simulink model "affine_single_integrator"  (R2020b)
settings: Solver=ode4  StartTime=0.0  StopTime=50  FixedStep=0.01  RelTol=1e-3
InitFcn:
  | Initial_Parameters;
values from neighbouring files (symbols this model uses):
  c_y = 0    [Initial_Parameters.m]
  delay = 0.01    [Initial_Parameters.m]    (also in run_by_script.m = 1)
  kalpha = 0.5    [Initial_Parameters.m]    (also in run_by_script.m = 4)
  kbeta = 1.5    [Initial_Parameters.m]    (also in run_by_script.m = 0.5)
  P0 = [2 0 ... (first row only)    [Initial_Parameters.m]    (also in run_by_script.m = [p(1,1:2:end)' p(2,2:2:end)'])
  stressMat = -fcn_StressMatrix(2,nodenum,m,P,neighborMat,fig_shape)    [Initial_Parameters.m]    (also in fcn_StressMatrix.m = -stressMat)
  vel_x = 0.1    [Initial_Parameters.m]
  vel_y = 0.5    [Initial_Parameters.m]
  w_y = 0.5    [Initial_Parameters.m]
settings Model: Creator=Fitz  LastModifiedBy=xpp
settings DebuggingCC: UnderSpecifiedDimensionMsg=warning

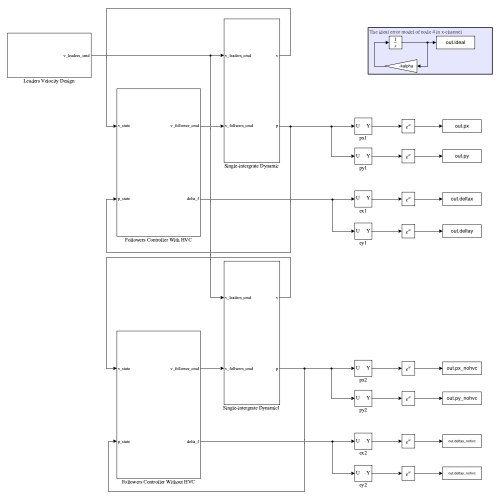
[thumbnail: Simulink's stored preview of the top-level diagram]
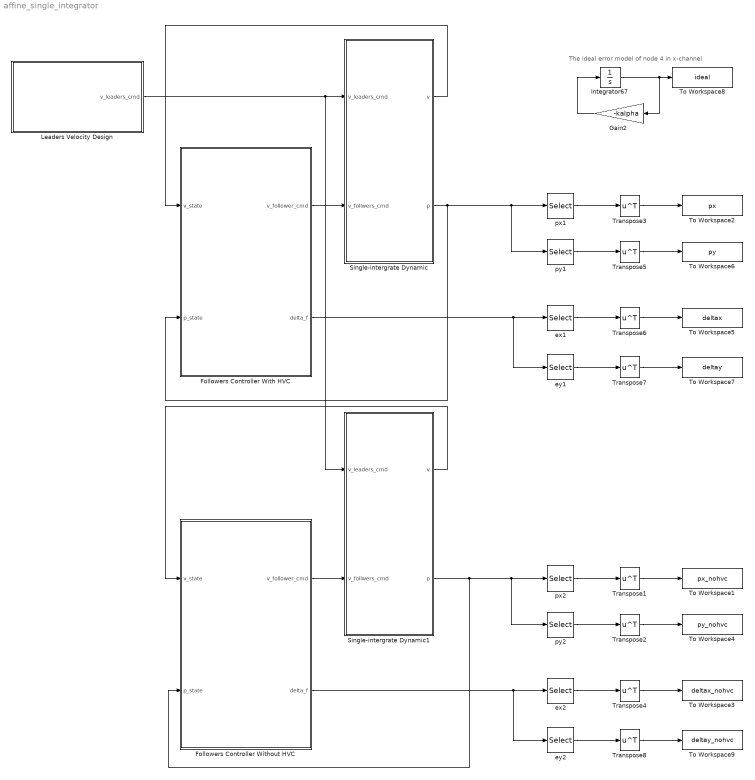
== system affine_single_integrator ==
  note: The ideal error model of node 4 in x-channel
  Followers Controller With HVC : Subsystem
  Followers Controller Without HVC : Subsystem
  Gain2 : Gain  Gain=-kalpha
  Integrator67 : Integrator  InitialCondition=P0(4,1)
  Leaders Velocity Design : Subsystem
  Single-intergrate Dynamic : Subsystem
  Single-intergrate Dynamic1 : Subsystem
  To Workspace1 : ToWorkspace  VariableName=px_nohvc  SampleTime=-1
      settings: Save2DSignal=2-D array (concatenate along first dimension)
  To Workspace2 : ToWorkspace  VariableName=px  SampleTime=-1
      settings: Save2DSignal=2-D array (concatenate along first dimension)
  To Workspace3 : ToWorkspace  VariableName=deltax_nohvc  SampleTime=-1
      settings: Save2DSignal=2-D array (concatenate along first dimension)
  To Workspace4 : ToWorkspace  VariableName=py_nohvc  SampleTime=-1
      settings: Save2DSignal=2-D array (concatenate along first dimension)
  To Workspace5 : ToWorkspace  VariableName=deltax  SampleTime=-1
      settings: Save2DSignal=2-D array (concatenate along first dimension)
  To Workspace6 : ToWorkspace  VariableName=py  SampleTime=-1
      settings: Save2DSignal=2-D array (concatenate along first dimension)
  To Workspace7 : ToWorkspace  VariableName=deltay  SampleTime=-1
      settings: Save2DSignal=2-D array (concatenate along first dimension)
  To Workspace8 : ToWorkspace  VariableName=ideal  SampleTime=-1
      settings: Save2DSignal=2-D array (concatenate along first dimension)
  To Workspace9 : ToWorkspace  VariableName=deltay_nohvc  SampleTime=-1
      settings: Save2DSignal=2-D array (concatenate along first dimension)
  Transpose{1..8} (8 alike) : Math  Operator=transpose  SaturateOnIntegerOverflow=on
  ex1 : Selector  NumberOfDimensions=2  InputPortWidth=3  IndexOptions=Select all,Index vector (dialog)  Indices=[1 3],1  OutputSizes=1,1
  ex2 : Selector  NumberOfDimensions=2  InputPortWidth=3  IndexOptions=Select all,Index vector (dialog)  Indices=[1 3],1  OutputSizes=1,1
  ey1 : Selector  NumberOfDimensions=2  InputPortWidth=3  IndexOptions=Select all,Index vector (dialog)  Indices=[1 3],2  OutputSizes=1,1
  ey2 : Selector  NumberOfDimensions=2  InputPortWidth=3  IndexOptions=Select all,Index vector (dialog)  Indices=[1 3],2  OutputSizes=1,1
  px1 : Selector  NumberOfDimensions=2  InputPortWidth=3  IndexOptions=Select all,Index vector (dialog)  Indices=[1 3],1  OutputSizes=1,1
  px2 : Selector  NumberOfDimensions=2  InputPortWidth=3  IndexOptions=Select all,Index vector (dialog)  Indices=[1 3],1  OutputSizes=1,1
  py1 : Selector  NumberOfDimensions=2  InputPortWidth=3  IndexOptions=Select all,Index vector (dialog)  Indices=[1 3],2  OutputSizes=1,1
  py2 : Selector  NumberOfDimensions=2  InputPortWidth=3  IndexOptions=Select all,Index vector (dialog)  Indices=[1 3],2  OutputSizes=1,1
  wires:
  Leaders Velocity Design/1(v_leaders_cmd) -> Single-intergrate Dynamic1/1(v_leaders_cmd), Single-intergrate Dynamic/1(v_leaders_cmd)
  Followers Controller With HVC/1(v_follower_cmd) -> Single-intergrate Dynamic/2(v_follwers_cmd)
  Single-intergrate Dynamic/1(v) -> Followers Controller With HVC/1(v_state)
  ey1/1 -> Transpose7/1
  py1/1 -> Transpose5/1
  Transpose3/1 -> To Workspace2/1
  Transpose7/1 -> To Workspace7/1
  Followers Controller With HVC/2(delta_f) -> ex1/1, ey1/1
  Transpose5/1 -> To Workspace6/1
  ex1/1 -> Transpose6/1
  Single-intergrate Dynamic/2(p) -> py1/1, px1/1, Followers Controller With HVC/2(p_state)
  Transpose6/1 -> To Workspace5/1
  px1/1 -> Transpose3/1
  Gain2/1 -> Integrator67/1
  Integrator67/1 -> To Workspace8/1, Gain2/1
  Followers Controller Without HVC/1(v_follower_cmd) -> Single-intergrate Dynamic1/2(v_follwers_cmd)
  Single-intergrate Dynamic1/1(v) -> Followers Controller Without HVC/1(v_state)
  Transpose1/1 -> To Workspace1/1
  ex2/1 -> Transpose4/1
  py2/1 -> Transpose2/1
  Followers Controller Without HVC/2(delta_f) -> ex2/1, ey2/1
  px2/1 -> Transpose1/1
  Transpose8/1 -> To Workspace9/1
  Transpose2/1 -> To Workspace4/1
  Transpose4/1 -> To Workspace3/1
  Single-intergrate Dynamic1/2(p) -> py2/1, px2/1, Followers Controller Without HVC/2(p_state)
  ey2/1 -> Transpose8/1

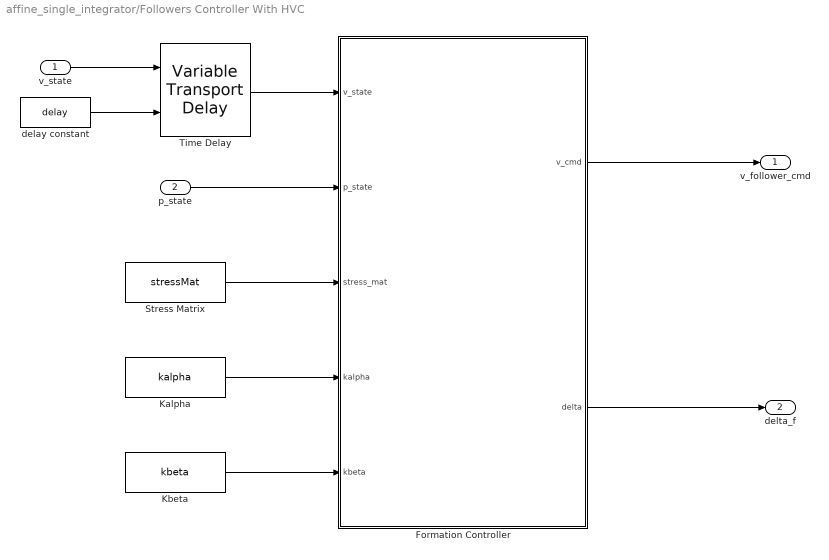
== system affine_single_integrator/Followers Controller With HVC ==
  v_state : Inport
  p_state : Inport  Port=2
  Formation Controller : MATLAB Function  TreatAsAtomicUnit=on
  Kalpha : Constant  Value=kalpha
  Kbeta : Constant  Value=kbeta
  Stress Matrix : Constant  Value=stressMat
  Time Delay : VariableTransportDelay  MaximumDelay=10
  delay constant : Constant  Value=delay
  v_follower_cmd : Outport
  delta_f : Outport  Port=2
  wires:
  delay constant/1 -> Time Delay/2
  v_state/1 -> Time Delay/1
  p_state/1 -> Formation Controller/2(p_state)
  Stress Matrix/1 -> Formation Controller/3(stress_mat)
  Kbeta/1 -> Formation Controller/5(kbeta)
  Kalpha/1 -> Formation Controller/4(kalpha)
  Formation Controller/1(v_cmd) -> v_follower_cmd/1
  Formation Controller/2(delta) -> delta_f/1
  Time Delay/1 -> Formation Controller/1(v_state)

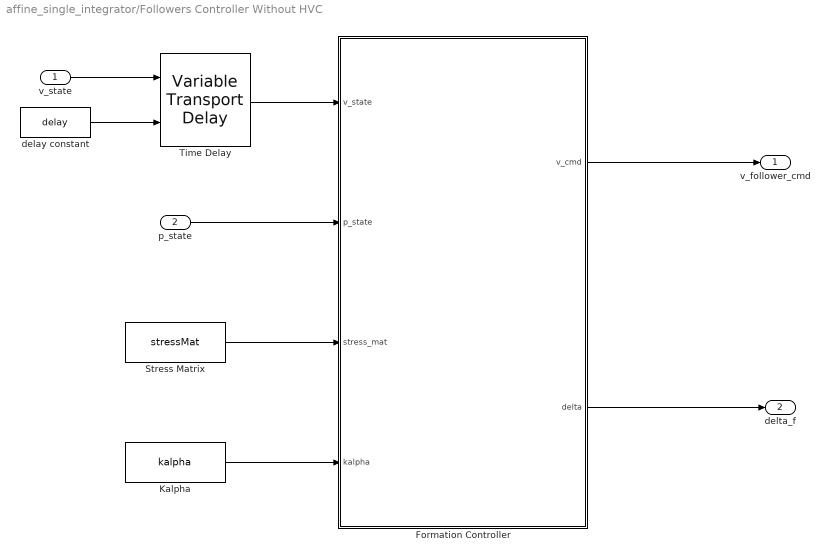
== system affine_single_integrator/Followers Controller Without HVC ==
  v_state : Inport
  p_state : Inport  Port=2
  Formation Controller : MATLAB Function  TreatAsAtomicUnit=on
  Kalpha : Constant  Value=kalpha
  Stress Matrix : Constant  Value=stressMat
  Time Delay : VariableTransportDelay  MaximumDelay=10
  delay constant : Constant  Value=delay
  v_follower_cmd : Outport
  delta_f : Outport  Port=2
  wires:
  delay constant/1 -> Time Delay/2
  v_state/1 -> Time Delay/1
  p_state/1 -> Formation Controller/2(p_state)
  Stress Matrix/1 -> Formation Controller/3(stress_mat)
  Kalpha/1 -> Formation Controller/4(kalpha)
  Formation Controller/1(v_cmd) -> v_follower_cmd/1
  Formation Controller/2(delta) -> delta_f/1
  Time Delay/1 -> Formation Controller/1(v_state)

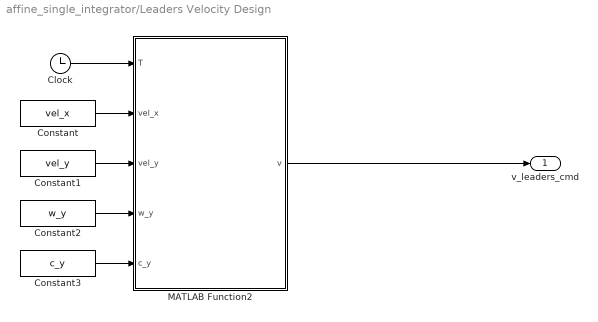
== system affine_single_integrator/Leaders Velocity Design ==
  Clock : Clock
  Constant : Constant  Value=vel_x
  Constant1 : Constant  Value=vel_y
  Constant2 : Constant  Value=w_y
  Constant3 : Constant  Value=c_y
  MATLAB Function2 : MATLAB Function  TreatAsAtomicUnit=on
  v_leaders_cmd : Outport
  wires:
  MATLAB Function2/1(v) -> v_leaders_cmd/1
  Clock/1 -> MATLAB Function2/1(T)
  Constant/1 -> MATLAB Function2/2(vel_x)
  Constant1/1 -> MATLAB Function2/3(vel_y)
  Constant2/1 -> MATLAB Function2/4(w_y)
  Constant3/1 -> MATLAB Function2/5(c_y)

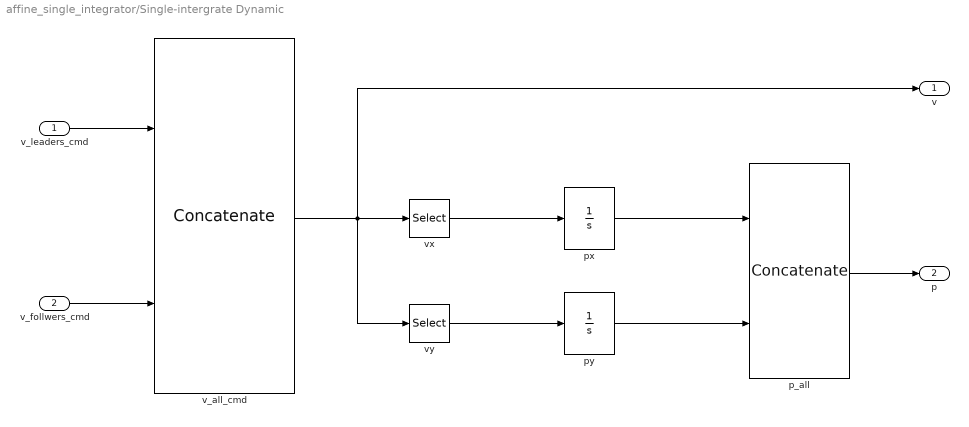
== system affine_single_integrator/Single-intergrate Dynamic ==
  v_leaders_cmd : Inport
  v_follwers_cmd : Inport  Port=2
  p_all : Concatenate  Mode=Multidimensional array  ConcatenateDimension=2
  px : Integrator  InitialCondition=P0(:,1)
  py : Integrator  InitialCondition=P0(:,2)
  v_all_cmd : Concatenate  Mode=Multidimensional array
  vx : Selector  NumberOfDimensions=2  InputPortWidth=3  IndexOptions=Select all,Index vector (dialog)  Indices=[1 3],1  OutputSizes=1,1
  vy : Selector  NumberOfDimensions=2  InputPortWidth=3  IndexOptions=Select all,Index vector (dialog)  Indices=[1 3],2  OutputSizes=1,1
  v : Outport
  p : Outport  Port=2
  wires:
  px/1 -> p_all/1
  py/1 -> p_all/2
  p_all/1 -> p/1
  v_leaders_cmd/1 -> v_all_cmd/1
  v_follwers_cmd/1 -> v_all_cmd/2
  v_all_cmd/1 -> vy/1, v/1, vx/1
  vx/1 -> px/1
  vy/1 -> py/1

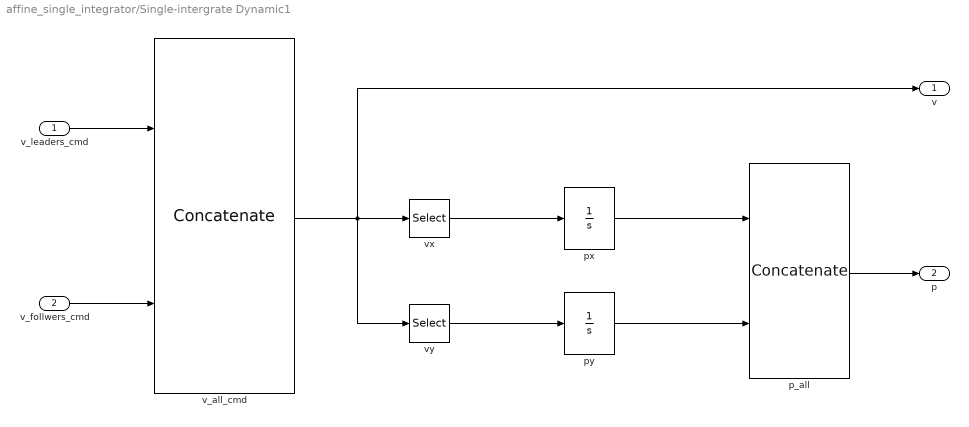
== system affine_single_integrator/Single-intergrate Dynamic1 ==
  v_leaders_cmd : Inport
  v_follwers_cmd : Inport  Port=2
  p_all : Concatenate  Mode=Multidimensional array  ConcatenateDimension=2
  px : Integrator  InitialCondition=P0(:,1)
  py : Integrator  InitialCondition=P0(:,2)
  v_all_cmd : Concatenate  Mode=Multidimensional array
  vx : Selector  NumberOfDimensions=2  InputPortWidth=3  IndexOptions=Select all,Index vector (dialog)  Indices=[1 3],1  OutputSizes=1,1
  vy : Selector  NumberOfDimensions=2  InputPortWidth=3  IndexOptions=Select all,Index vector (dialog)  Indices=[1 3],2  OutputSizes=1,1
  v : Outport
  p : Outport  Port=2
  wires:
  px/1 -> p_all/1
  py/1 -> p_all/2
  p_all/1 -> p/1
  v_leaders_cmd/1 -> v_all_cmd/1
  v_follwers_cmd/1 -> v_all_cmd/2
  v_all_cmd/1 -> vy/1, v/1, vx/1
  vx/1 -> px/1
  vy/1 -> py/1

== matlab function affine_single_integrator/Followers Controller With HVC/Formation Controller ==
  data: v_state input; p_state input; stress_mat input; kalpha input; v_cmd output size=[followerNum, dim]; kbeta input; delta output
function [v_cmd, delta] = formation_controller(v_state, p_state, stress_mat, kalpha, kbeta)
leaders_num = 3;
stressmat_ff = stress_mat(leaders_num+1:end,leaders_num+1:end);
stressmat_fl = stress_mat(leaders_num+1:end,1:leaders_num);
inv_stressmat_ff = inv(stressmat_ff);

delta = p_state(leaders_num+1:end,:) + inv_stressmat_ff * stressmat_fl * p_state(1:leaders_num,:);
E = stressmat_fl * p_state(1:leaders_num,:) + stressmat_ff * p_state(leaders_num+1:end,:);
dE = stressmat_fl * v_state(1:leaders_num,:) + stressmat_ff * v_state(leaders_num+1:end,:);

v_cmd = v_state(leaders_num+1:end,:) - kbeta * (kalpha*E + dE);

== matlab function affine_single_integrator/Followers Controller Without HVC/Formation Controller ==
  data: v_state input; p_state input; stress_mat input; kalpha input; v_cmd output size=[followerNum, dim]; delta output
function [v_cmd, delta] = formation_controller(v_state, p_state, stress_mat, kalpha)
leaders_num = 3;
stressmat_ff = stress_mat(leaders_num+1:end,leaders_num+1:end);
stressmat_fl = stress_mat(leaders_num+1:end,1:leaders_num);
inv_stressmat_ff = inv(stressmat_ff);

delta = p_state(leaders_num+1:end,:) + inv_stressmat_ff * stressmat_fl * p_state(1:leaders_num,:);
E = stressmat_fl * p_state(1:leaders_num,:) + stressmat_ff * p_state(leaders_num+1:end,:);
ki = diag(stress_mat);
ki = ki(leaders_num+1:end);

% stress_new = -stress_mat;
% for i = 1:size(stress_new, 1)
%     stress_new(i,i) = 0;
% end

%v_cmd = kalpha*E - stress_new(leaders_num+1,:)*v_state;
v_cmd = kalpha*E;
for i = 1:length(ki)
    % v_cmd(i,:) = v_cmd(i,:) - sum([stress_mat(i+leaders_num,:); stress_mat(i+leaders_num,:)]'.*v_state, 1);
    for j = 1:size(stress_mat, 1)
        if j == (i+leaders_num)
            continue;
        end
        wij = -stress_mat(i+leaders_num,j);
        v_cmd(i,:) = v_cmd(i,:) - wij*v_state(j,:);
    end
    v_cmd(i,:) = -v_cmd(i,:)./ki(i);
end

== matlab function affine_single_integrator/Leaders Velocity Design/MATLAB Function2 ==
  data: T input; v output; vel_x input; vel_y input; w_y input; c_y input
function v = fcn_leaderV(T,vel_x,vel_y,w_y,c_y)
leaders_num = 3;
v = zeros(leaders_num, 2);
current_time = T;

%% cos signal
vx = vel_x;
vy = vel_y*cos(w_y*current_time)+c_y;

v(:,1) = ones(leaders_num, 1) * vx;
v(:,2) = ones(leaders_num, 1) * vy;
end
